simulink model "fourBebop_circle"  (R2017b)
settings: Solver=FixedStepAuto  StartTime=0.0  StopTime=inf  FixedStep=sampleTime  RelTol=1e-3  EnableMultiTasking=on
undefined symbols (not defined in the file or in its folder): Angular, Linear, R
libraries: simulink x20, robotlib x20
(part 1 of 2)
settings Model: Creator=exbot  LastModifiedBy=root
settings DataIOCC: LimitDataPoints=on
settings OptimizationCC: LifeSpan=inf  MaxStackSize=64
settings DebuggingCC: ParameterTunabilityLossMsg=error  AllowSymbolicDim=off  SFUnexpectedBacktrackingDiag=warning  SFNoUnconditionalDefaultTransitionDiag=warning  SFExecutionAtInitializationDiag=none
settings HardwareCC: ProdBitPerPointer=32  ProdBitPerSizeT=32  ProdBitPerPtrDiffT=32  ProdLargestAtomicFloat=None  ProdIntDivRoundTo=Undefined  ProdEndianess=Unspecified  ProdWordSize=32  ProdHWDeviceType=Generic->Unspecified (assume 32-bit Generic)
settings ModelReferenceCC: PropagateSignalLabelsOutOfModel=off
settings SFSimCC: MATLABDynamicMemAlloc=off
settings RTWCC: SystemTargetFile=ert.tlc  HardwareBoard=Robot Operating System (ROS)  TemplateMakefile=ert_default_tmf  Toolchain=Catkin  TargetLang=C++
settings CodeAppCC: ForceParamTrailComments=on  IgnoreCustomStorageClasses=off  OperatorAnnotations=on  SimulinkDataObjDesc=on  SFDataObjDesc=on  MATLABFcnDesc=on  InsertBlockDesc=on  StateflowObjectComments=on  MATLABSourceComments=on
settings ERTTargetCC: MultiwordLength=2048  SupportContinuousTime=on
settings ConfigComp: CovMetricSettings=dw  CovHtmlReporting=on  CovSaveCumulativeToWorkspaceVar=on  CovSaveSingleToWorkspaceVar=on  CovExternalEMLEnable=off

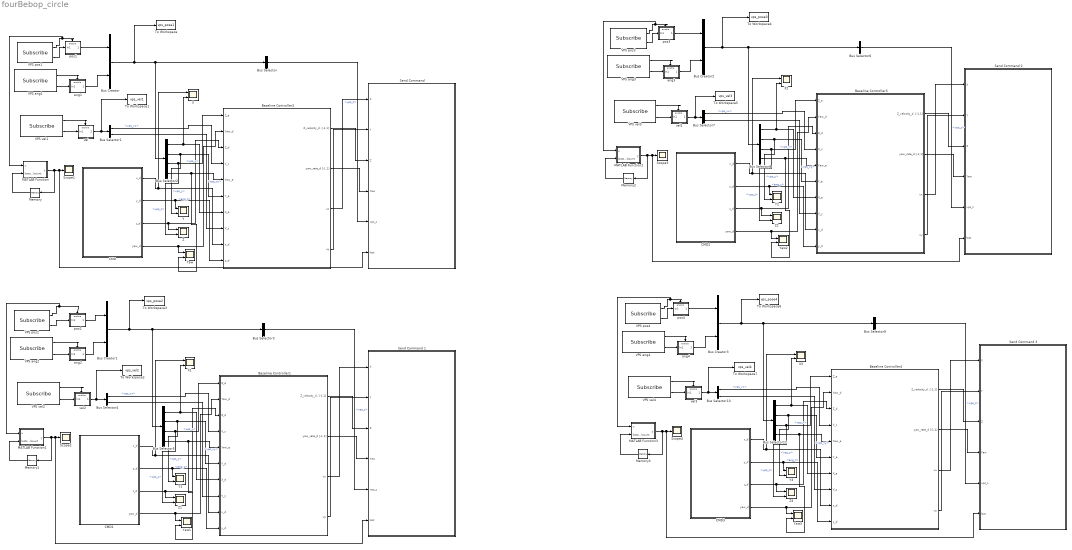
== system fourBebop_circle ==
  Baseline Controller1 : Subsystem  AncestorBlock=ARBlocks/Baseline Controller
  Baseline Controller2 : Subsystem  AncestorBlock=ARBlocks/Baseline Controller
  Baseline Controller3 : Subsystem  AncestorBlock=ARBlocks/Baseline Controller
  Baseline Controller4 : Subsystem  AncestorBlock=ARBlocks/Baseline Controller
  Bus Creator{,1..3} (4 alike) : BusCreator  Inputs=2
  Bus Selector{,3,6,9} (4 alike) : BusSelector  OutputSignals=signal1.vps_z
  Bus Selector{1,4,7,10} (4 alike) : BusSelector  OutputSignals=vps_vx,vps_vy
  Bus Selector{2,5,8,11} (4 alike) : BusSelector  OutputSignals=signal1.vps_x,signal1.vps_y,signal1.vps_z,signal2.ang_z
  CMD : Subsystem
  CMD1 : Subsystem
  CMD2 : Subsystem
  CMD3 : Subsystem
  MATLAB Function : MATLAB Function  TreatAsAtomicUnit=on
  MATLAB Function1 : MATLAB Function  TreatAsAtomicUnit=on
  MATLAB Function2 : MATLAB Function  TreatAsAtomicUnit=on
  MATLAB Function3 : MATLAB Function  TreatAsAtomicUnit=on
  Memory{,1..3} (4 alike) : Memory
  Scope{1..4} (4 alike) : Scope
  "Send Command " : Subsystem
  Send Command 1 : Subsystem
  Send Command 2 : Subsystem
  Send Command 3 : Subsystem
  To Workspace : ToWorkspace  VariableName=vps_pose1  SaveFormat=Timeseries  SampleTime=-1
  To Workspace1 : ToWorkspace  VariableName=vps_vel1  SaveFormat=Timeseries  SampleTime=-1
  To Workspace2 : ToWorkspace  VariableName=vps_vel2  SaveFormat=Timeseries  SampleTime=-1
  To Workspace3 : ToWorkspace  VariableName=vps_pose2  SaveFormat=Timeseries  SampleTime=-1
  To Workspace4 : ToWorkspace  VariableName=vps_pose3  SaveFormat=Timeseries  SampleTime=-1
  To Workspace5 : ToWorkspace  VariableName=vps_vel3  SaveFormat=Timeseries  SampleTime=-1
  To Workspace6 : ToWorkspace  VariableName=vps_pose4  SaveFormat=Timeseries  SampleTime=-1
  To Workspace7 : ToWorkspace  VariableName=vps_vel4  SaveFormat=Timeseries  SampleTime=-1
  VPS ang1 : robotlib/Subscribe  SourceLibraryInfo=This block requires Robotics System Toolbox  topicSource=Select from ROS network  topic=/vps_ang1  messageType=geometry_msgs/PointStamped  sampleTime=-1  messageQueueLength=1
      settings: SourceProductBaseCode=RO
  VPS ang2 : robotlib/Subscribe  SourceLibraryInfo=This block requires Robotics System Toolbox  topicSource=Specify your own  topic=/vps_ang2  messageType=geometry_msgs/PointStamped  sampleTime=-1  messageQueueLength=1
      settings: SourceProductBaseCode=RO
  VPS ang3 : robotlib/Subscribe  SourceLibraryInfo=This block requires Robotics System Toolbox  topicSource=Specify your own  topic=/vps_ang3  messageType=geometry_msgs/PointStamped  sampleTime=-1  messageQueueLength=1
      settings: SourceProductBaseCode=RO
  VPS ang4 : robotlib/Subscribe  SourceLibraryInfo=This block requires Robotics System Toolbox  topicSource=Specify your own  topic=/vps_ang4  messageType=geometry_msgs/PointStamped  sampleTime=-1  messageQueueLength=1
      settings: SourceProductBaseCode=RO
  VPS pos1 : robotlib/Subscribe  SourceLibraryInfo=This block requires Robotics System Toolbox  topicSource=Select from ROS network  topic=/vps_pos1  messageType=geometry_msgs/PointStamped  sampleTime=-1  messageQueueLength=1
      settings: SourceProductBaseCode=RO
  VPS pos2 : robotlib/Subscribe  SourceLibraryInfo=This block requires Robotics System Toolbox  topicSource=Specify your own  topic=/vps_pos2  messageType=geometry_msgs/PointStamped  sampleTime=-1  messageQueueLength=1
      settings: SourceProductBaseCode=RO
  VPS pos3 : robotlib/Subscribe  SourceLibraryInfo=This block requires Robotics System Toolbox  topicSource=Specify your own  topic=/vps_pos3  messageType=geometry_msgs/PointStamped  sampleTime=-1  messageQueueLength=1
      settings: SourceProductBaseCode=RO
  VPS pos4 : robotlib/Subscribe  SourceLibraryInfo=This block requires Robotics System Toolbox  topicSource=Specify your own  topic=/vps_pos4  messageType=geometry_msgs/PointStamped  sampleTime=-1  messageQueueLength=1
      settings: SourceProductBaseCode=RO
  VPS vel1 : robotlib/Subscribe  SourceLibraryInfo=This block requires Robotics System Toolbox  topicSource=Select from ROS network  topic=/vps_vel1  messageType=geometry_msgs/TwistStamped  sampleTime=-1  messageQueueLength=1
      settings: SourceProductBaseCode=RO
  VPS vel2 : robotlib/Subscribe  SourceLibraryInfo=This block requires Robotics System Toolbox  topicSource=Specify your own  topic=/vps_vel2  messageType=geometry_msgs/TwistStamped  sampleTime=-1  messageQueueLength=1
      settings: SourceProductBaseCode=RO
  VPS vel3 : robotlib/Subscribe  SourceLibraryInfo=This block requires Robotics System Toolbox  topicSource=Specify your own  topic=/vps_vel3  messageType=geometry_msgs/TwistStamped  sampleTime=-1  messageQueueLength=1
      settings: SourceProductBaseCode=RO
  VPS vel4 : robotlib/Subscribe  SourceLibraryInfo=This block requires Robotics System Toolbox  topicSource=Specify your own  topic=/vps_vel4  messageType=geometry_msgs/TwistStamped  sampleTime=-1  messageQueueLength=1
      settings: SourceProductBaseCode=RO
  X{,1..3} (4 alike) : Scope  NumInputPorts=2
  Y{,1..3} (4 alike) : Scope  NumInputPorts=2
  Yaw{,1..3} (4 alike) : Scope  NumInputPorts=2
  Z{,1..3} (4 alike) : Scope  NumInputPorts=2
  ang1 : Subsystem
  ang2 : Subsystem
  ang3 : Subsystem
  ang4 : Subsystem
  pos1 : Subsystem
  pos2 : Subsystem
  pos3 : Subsystem
  pos4 : Subsystem
  vel : Subsystem
  vel1 : Subsystem
  vel2 : Subsystem
  vel3 : Subsystem
  wires:
  Bus Creator/1 -> To Workspace/1, Bus Selector2/1, Bus Selector/1
  vel/1(Out1) -> To Workspace1/1, Bus Selector1/1
  Baseline Controller2/3(ux) -> "Send Command "/1(X)
  Baseline Controller2/4(uy) -> "Send Command "/2(Y)
  Baseline Controller2/1(Z_velocity_d. [-1,1]) -> "Send Command "/3(Z)
  Baseline Controller2/2(yaw_rate_d [-1,1]) -> "Send Command "/4(Yaw)
  VPS ang1/1 -> ang1/Enable
  pos1/1(Out1) -> Bus Creator/1
  VPS ang1/2 -> ang1/1(In1)
  VPS pos1/2 -> pos1/1(In1)
  ang1/1(Out1) -> Bus Creator/2
  VPS vel1/1 -> vel/Enable
  VPS vel1/2 -> vel/1(In1)
  Bus Selector/1 -> "Send Command "/5(vps_z)  "<vps_z>"
  Memory/1 -> MATLAB Function/2(lostsigalcount)
  VPS pos1/1 -> MATLAB Function/1(u), pos1/Enable
  MATLAB Function/1(y) -> Memory/1, "Send Command "/6(lost), Scope1/1
  Bus Selector1/1 -> Baseline Controller2/4(" V_x")  "<vps_vx>"
  Bus Selector1/2 -> Baseline Controller2/8(V_y)  "<vps_vy>"
  Bus Selector2/4 -> Yaw/2, Baseline Controller2/5(Yaw_e)  "<ang_z>"
  Bus Selector2/1 -> X/2, Baseline Controller2/7(X_e)  "<vps_x>"
  Bus Selector2/2 -> Y/2, Baseline Controller2/6(Y_e)  "<vps_y>"
  Bus Selector2/3 -> Z/2, Baseline Controller2/1(" Z_e ")  "<vps_z>"
  CMD/4(yaw_d) -> Yaw/1, Baseline Controller2/2(Yaw_d)
  CMD/3(z_d) -> Z/1, Baseline Controller2/3(Z_d)
  CMD/2(y_d) -> Y/1, Baseline Controller2/10(y_d)
  CMD/1(x_d) -> X/1, Baseline Controller2/9(x_d)
  VPS pos2/1 -> MATLAB Function1/1(u), pos2/Enable
  Bus Selector5/2 -> Y1/2, Baseline Controller1/6(Y_e)  "<vps_y>"
  CMD1/1(x_d) -> X1/1, Baseline Controller1/9(x_d)
  Bus Selector3/1 -> Send Command 1/5(vps_z)  "<vps_z>"
  CMD1/2(y_d) -> Y1/1, Baseline Controller1/10(y_d)
  ang2/1(Out1) -> Bus Creator1/2
  Bus Selector5/1 -> X1/2, Baseline Controller1/7(X_e)  "<vps_x>"
  Baseline Controller1/4(uy) -> Send Command 1/2(Y)
  VPS ang2/1 -> ang2/Enable
  Baseline Controller1/2(yaw_rate_d [-1,1]) -> Send Command 1/4(Yaw)
  VPS pos2/2 -> pos2/1(In1)
  vel2/1(Out1) -> To Workspace2/1, Bus Selector4/1
  Bus Selector4/1 -> Baseline Controller1/4(" V_x")  "<vps_vx>"
  Bus Selector4/2 -> Baseline Controller1/8(V_y)  "<vps_vy>"
  Bus Selector5/3 -> Z1/2, Baseline Controller1/1(" Z_e ")  "<vps_z>"
  CMD1/4(yaw_d) -> Yaw1/1, Baseline Controller1/2(Yaw_d)
  pos2/1(Out1) -> Bus Creator1/1
  VPS vel2/2 -> vel2/1(In1)
  VPS vel2/1 -> vel2/Enable
  Bus Creator1/1 -> To Workspace3/1, Bus Selector5/1, Bus Selector3/1
  Bus Selector5/4 -> Yaw1/2, Baseline Controller1/5(Yaw_e)  "<ang_z>"
  VPS ang2/2 -> ang2/1(In1)
  Baseline Controller1/3(ux) -> Send Command 1/1(X)
  Baseline Controller1/1(Z_velocity_d. [-1,1]) -> Send Command 1/3(Z)
  CMD1/3(z_d) -> Z1/1, Baseline Controller1/3(Z_d)
  MATLAB Function1/1(y) -> Memory1/1, Send Command 1/6(lost), Scope2/1
  Memory1/1 -> MATLAB Function1/2(lostsigalcount)
  VPS pos3/1 -> MATLAB Function2/1(u), pos3/Enable
  VPS ang3/2 -> ang3/1(In1)
  Bus Selector6/1 -> Send Command 2/5(vps_z)  "<vps_z>"
  pos3/1(Out1) -> Bus Creator2/1
  Bus Selector7/1 -> Baseline Controller3/4(" V_x")  "<vps_vx>"
  Bus Selector8/4 -> Yaw2/2, Baseline Controller3/5(Yaw_e)  "<ang_z>"
  vel1/1(Out1) -> To Workspace5/1, Bus Selector7/1
  Bus Selector8/3 -> Z2/2, Baseline Controller3/1(" Z_e ")  "<vps_z>"
  VPS pos3/2 -> pos3/1(In1)
  Baseline Controller3/2(yaw_rate_d [-1,1]) -> Send Command 2/4(Yaw)
  CMD2/3(z_d) -> Z2/1, Baseline Controller3/3(Z_d)
  Baseline Controller3/4(uy) -> Send Command 2/2(Y)
  Memory2/1 -> MATLAB Function2/2(lostsigalcount)
  Bus Selector8/1 -> X2/2, Baseline Controller3/7(X_e)  "<vps_x>"
  Bus Creator2/1 -> To Workspace4/1, Bus Selector8/1, Bus Selector6/1
  CMD2/2(y_d) -> Y2/1, Baseline Controller3/10(y_d)
  Bus Selector7/2 -> Baseline Controller3/8(V_y)  "<vps_vy>"
  VPS ang3/1 -> ang3/Enable
  Baseline Controller3/3(ux) -> Send Command 2/1(X)
  Baseline Controller3/1(Z_velocity_d. [-1,1]) -> Send Command 2/3(Z)
  VPS vel3/2 -> vel1/1(In1)
  VPS vel3/1 -> vel1/Enable
  ang3/1(Out1) -> Bus Creator2/2
  MATLAB Function2/1(y) -> Memory2/1, Send Command 2/6(lost), Scope3/1
  CMD2/4(yaw_d) -> Yaw2/1, Baseline Controller3/2(Yaw_d)
  CMD2/1(x_d) -> X2/1, Baseline Controller3/9(x_d)
  Bus Selector8/2 -> Y2/2, Baseline Controller3/6(Y_e)  "<vps_y>"
  Bus Selector10/1 -> Baseline Controller4/4(" V_x")  "<vps_vx>"
  VPS vel4/2 -> vel3/1(In1)
  CMD3/3(z_d) -> Z3/1, Baseline Controller4/3(Z_d)
  Bus Creator3/1 -> To Workspace6/1, Bus Selector11/1, Bus Selector9/1
  Bus Selector11/4 -> Yaw3/2, Baseline Controller4/5(Yaw_e)  "<ang_z>"
  CMD3/4(yaw_d) -> Yaw3/1, Baseline Controller4/2(Yaw_d)
  VPS pos4/1 -> MATLAB Function3/1(u), pos4/Enable
  Baseline Controller4/2(yaw_rate_d [-1,1]) -> Send Command 3/4(Yaw)
  Baseline Controller4/1(Z_velocity_d. [-1,1]) -> Send Command 3/3(Z)
  Bus Selector10/2 -> Baseline Controller4/8(V_y)  "<vps_vy>"
  ang4/1(Out1) -> Bus Creator3/2
  VPS pos4/2 -> pos4/1(In1)
  Memory3/1 -> MATLAB Function3/2(lostsigalcount)
  Baseline Controller4/3(ux) -> Send Command 3/1(X)
  Bus Selector11/1 -> X3/2, Baseline Controller4/7(X_e)  "<vps_x>"
  MATLAB Function3/1(y) -> Memory3/1, Send Command 3/6(lost), Scope4/1
  VPS vel4/1 -> vel3/Enable
  CMD3/2(y_d) -> Y3/1, Baseline Controller4/10(y_d)
  Bus Selector11/2 -> Y3/2, Baseline Controller4/6(Y_e)  "<vps_y>"
  Bus Selector11/3 -> Z3/2, Baseline Controller4/1(" Z_e ")  "<vps_z>"
  Baseline Controller4/4(uy) -> Send Command 3/2(Y)
  VPS ang4/2 -> ang4/1(In1)
  vel3/1(Out1) -> To Workspace7/1, Bus Selector10/1
  VPS ang4/1 -> ang4/Enable
  pos4/1(Out1) -> Bus Creator3/1
  CMD3/1(x_d) -> X3/1, Baseline Controller4/9(x_d)
  Bus Selector9/1 -> Send Command 3/5(vps_z)  "<vps_z>"

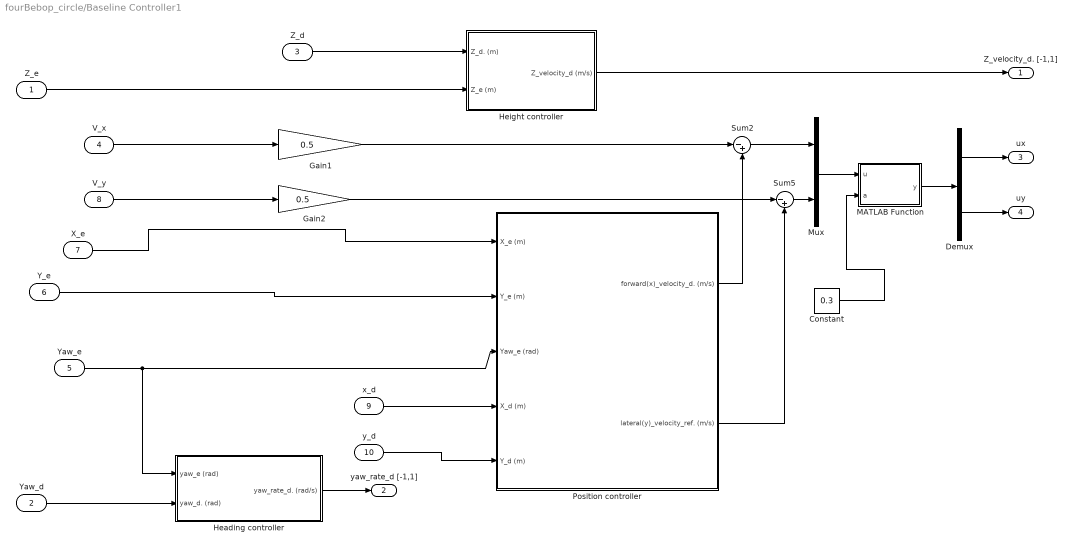
== system fourBebop_circle/Baseline Controller1 ==
  " Z_e " : Inport
  Yaw_d : Inport  Port=2
  Z_d : Inport  Port=3
  " V_x" : Inport  Port=4
  Yaw_e : Inport  Port=5
  Y_e : Inport  Port=6
  X_e : Inport  Port=7
  V_y : Inport  Port=8
  x_d : Inport  Port=9
  y_d : Inport  Port=10
  Constant : Constant  Value=0.3
  Demux : Demux  Outputs=2
  Gain1 : Gain  Gain=0.5
  Gain2 : Gain  Gain=0.5
  Heading controller : Subsystem
  "Height controller " : Subsystem
  MATLAB Function : MATLAB Function  TreatAsAtomicUnit=on
  Mux : Mux  Inputs=2
  Position controller : Subsystem
  Sum2 : Sum  Inputs=|-+
  Sum5 : Sum  Inputs=|-+
  Z_velocity_d. [-1,1] : Outport
  yaw_rate_d [-1,1] : Outport  Port=2
  ux : Outport  Port=3
  uy : Outport  Port=4
  wires:
  Position controller/2(lateral(y)_velocity_ref. (m/s)) -> Sum5/2
  Gain2/1 -> Sum5/1
  V_y/1 -> Gain2/1
  Position controller/1(forward(x)_velocity_d. (m/s)) -> Sum2/2
  Gain1/1 -> Sum2/1
  Yaw_e/1 -> Heading controller/1(yaw_e (rad)), Position controller/3(Yaw_e (rad))
  " Z_e "/1 -> "Height controller "/2(Z_e (m))
  "Height controller "/1(Z_velocity_d (m/s)) -> Z_velocity_d. [-1,1]/1
  " V_x"/1 -> Gain1/1
  Heading controller/1(yaw_rate_d. (rad/s)) -> yaw_rate_d [-1,1]/1
  X_e/1 -> Position controller/1(X_e (m))
  Y_e/1 -> Position controller/2(Y_e (m))
  Sum2/1 -> Mux/1
  Sum5/1 -> Mux/2
  Yaw_d/1 -> Heading controller/2(yaw_d. (rad))
  Mux/1 -> MATLAB Function/1(u)
  MATLAB Function/1(y) -> Demux/1
  Demux/1 -> ux/1
  Demux/2 -> uy/1
  Constant/1 -> MATLAB Function/2(a)
  Z_d/1 -> "Height controller "/1(Z_d. (m))
  x_d/1 -> Position controller/4(X_d (m))
  y_d/1 -> Position controller/5(Y_d (m))

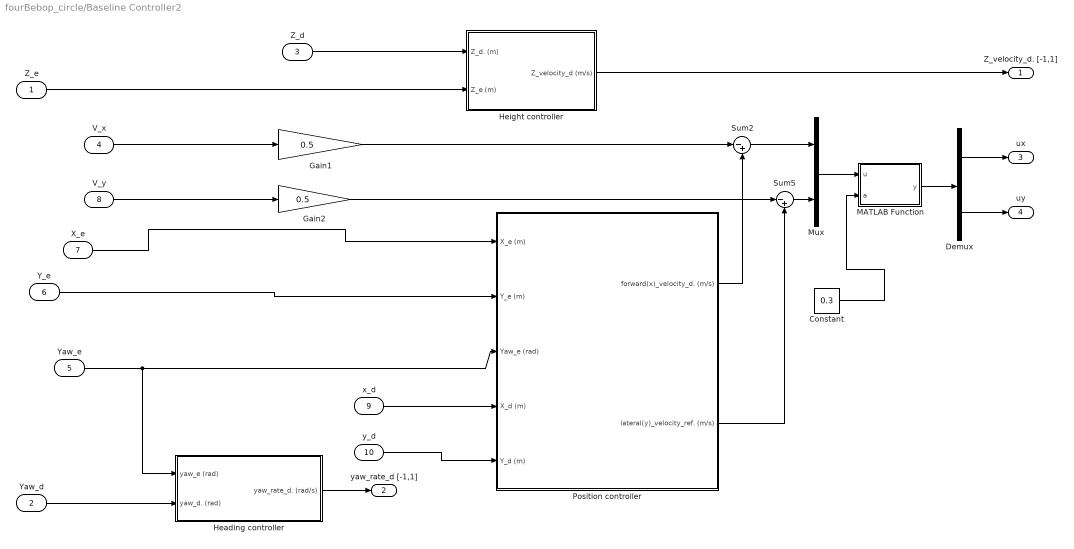
== system fourBebop_circle/Baseline Controller2 ==
  " Z_e " : Inport
  Yaw_d : Inport  Port=2
  Z_d : Inport  Port=3
  " V_x" : Inport  Port=4
  Yaw_e : Inport  Port=5
  Y_e : Inport  Port=6
  X_e : Inport  Port=7
  V_y : Inport  Port=8
  x_d : Inport  Port=9
  y_d : Inport  Port=10
  Constant : Constant  Value=0.3
  Demux : Demux  Outputs=2
  Gain1 : Gain  Gain=0.5
  Gain2 : Gain  Gain=0.5
  Heading controller : Subsystem
  "Height controller " : Subsystem
  MATLAB Function : MATLAB Function  TreatAsAtomicUnit=on
  Mux : Mux  Inputs=2
  Position controller : Subsystem
  Sum2 : Sum  Inputs=|-+
  Sum5 : Sum  Inputs=|-+
  Z_velocity_d. [-1,1] : Outport
  yaw_rate_d [-1,1] : Outport  Port=2
  ux : Outport  Port=3
  uy : Outport  Port=4
  wires:
  Position controller/2(lateral(y)_velocity_ref. (m/s)) -> Sum5/2
  Gain2/1 -> Sum5/1
  V_y/1 -> Gain2/1
  Position controller/1(forward(x)_velocity_d. (m/s)) -> Sum2/2
  Gain1/1 -> Sum2/1
  Yaw_e/1 -> Heading controller/1(yaw_e (rad)), Position controller/3(Yaw_e (rad))
  " Z_e "/1 -> "Height controller "/2(Z_e (m))
  "Height controller "/1(Z_velocity_d (m/s)) -> Z_velocity_d. [-1,1]/1
  " V_x"/1 -> Gain1/1
  Heading controller/1(yaw_rate_d. (rad/s)) -> yaw_rate_d [-1,1]/1
  X_e/1 -> Position controller/1(X_e (m))
  Y_e/1 -> Position controller/2(Y_e (m))
  Sum2/1 -> Mux/1
  Sum5/1 -> Mux/2
  Yaw_d/1 -> Heading controller/2(yaw_d. (rad))
  Mux/1 -> MATLAB Function/1(u)
  MATLAB Function/1(y) -> Demux/1
  Demux/1 -> ux/1
  Demux/2 -> uy/1
  Constant/1 -> MATLAB Function/2(a)
  Z_d/1 -> "Height controller "/1(Z_d. (m))
  x_d/1 -> Position controller/4(X_d (m))
  y_d/1 -> Position controller/5(Y_d (m))

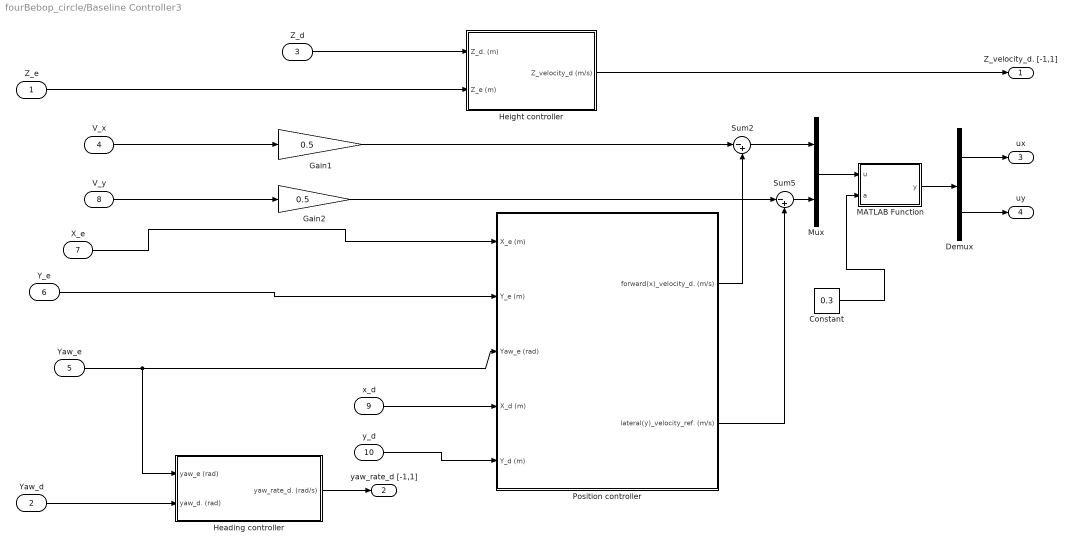
== system fourBebop_circle/Baseline Controller3 ==
  " Z_e " : Inport
  Yaw_d : Inport  Port=2
  Z_d : Inport  Port=3
  " V_x" : Inport  Port=4
  Yaw_e : Inport  Port=5
  Y_e : Inport  Port=6
  X_e : Inport  Port=7
  V_y : Inport  Port=8
  x_d : Inport  Port=9
  y_d : Inport  Port=10
  Constant : Constant  Value=0.3
  Demux : Demux  Outputs=2
  Gain1 : Gain  Gain=0.5
  Gain2 : Gain  Gain=0.5
  Heading controller : Subsystem
  "Height controller " : Subsystem
  MATLAB Function : MATLAB Function  TreatAsAtomicUnit=on
  Mux : Mux  Inputs=2
  Position controller : Subsystem
  Sum2 : Sum  Inputs=|-+
  Sum5 : Sum  Inputs=|-+
  Z_velocity_d. [-1,1] : Outport
  yaw_rate_d [-1,1] : Outport  Port=2
  ux : Outport  Port=3
  uy : Outport  Port=4
  wires:
  Position controller/2(lateral(y)_velocity_ref. (m/s)) -> Sum5/2
  Gain2/1 -> Sum5/1
  V_y/1 -> Gain2/1
  Position controller/1(forward(x)_velocity_d. (m/s)) -> Sum2/2
  Gain1/1 -> Sum2/1
  Yaw_e/1 -> Heading controller/1(yaw_e (rad)), Position controller/3(Yaw_e (rad))
  " Z_e "/1 -> "Height controller "/2(Z_e (m))
  "Height controller "/1(Z_velocity_d (m/s)) -> Z_velocity_d. [-1,1]/1
  " V_x"/1 -> Gain1/1
  Heading controller/1(yaw_rate_d. (rad/s)) -> yaw_rate_d [-1,1]/1
  X_e/1 -> Position controller/1(X_e (m))
  Y_e/1 -> Position controller/2(Y_e (m))
  Sum2/1 -> Mux/1
  Sum5/1 -> Mux/2
  Yaw_d/1 -> Heading controller/2(yaw_d. (rad))
  Mux/1 -> MATLAB Function/1(u)
  MATLAB Function/1(y) -> Demux/1
  Demux/1 -> ux/1
  Demux/2 -> uy/1
  Constant/1 -> MATLAB Function/2(a)
  Z_d/1 -> "Height controller "/1(Z_d. (m))
  x_d/1 -> Position controller/4(X_d (m))
  y_d/1 -> Position controller/5(Y_d (m))

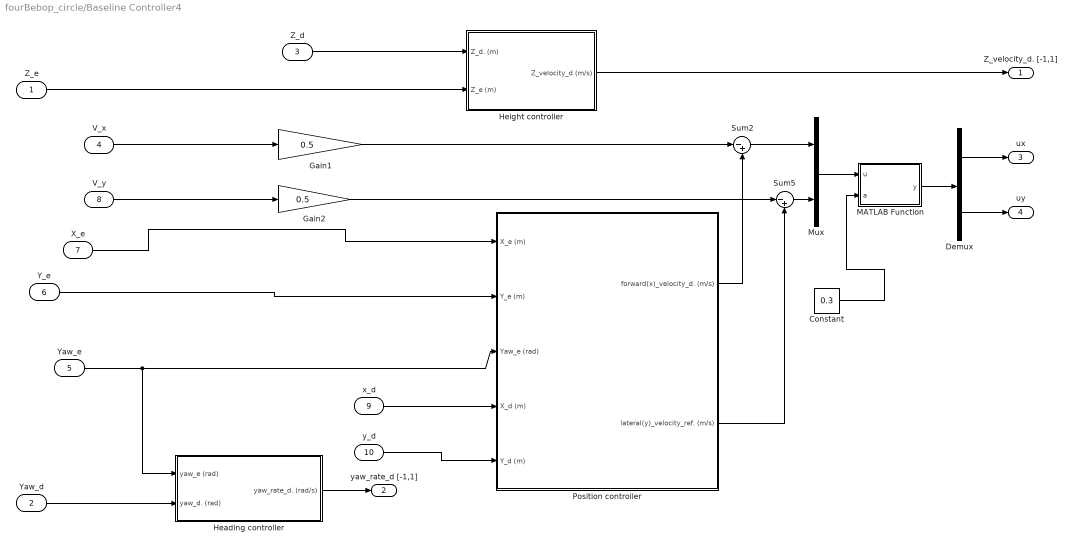
== system fourBebop_circle/Baseline Controller4 ==
  " Z_e " : Inport
  Yaw_d : Inport  Port=2
  Z_d : Inport  Port=3
  " V_x" : Inport  Port=4
  Yaw_e : Inport  Port=5
  Y_e : Inport  Port=6
  X_e : Inport  Port=7
  V_y : Inport  Port=8
  x_d : Inport  Port=9
  y_d : Inport  Port=10
  Constant : Constant  Value=0.3
  Demux : Demux  Outputs=2
  Gain1 : Gain  Gain=0.5
  Gain2 : Gain  Gain=0.5
  Heading controller : Subsystem
  "Height controller " : Subsystem
  MATLAB Function : MATLAB Function  TreatAsAtomicUnit=on
  Mux : Mux  Inputs=2
  Position controller : Subsystem
  Sum2 : Sum  Inputs=|-+
  Sum5 : Sum  Inputs=|-+
  Z_velocity_d. [-1,1] : Outport
  yaw_rate_d [-1,1] : Outport  Port=2
  ux : Outport  Port=3
  uy : Outport  Port=4
  wires:
  Position controller/2(lateral(y)_velocity_ref. (m/s)) -> Sum5/2
  Gain2/1 -> Sum5/1
  V_y/1 -> Gain2/1
  Position controller/1(forward(x)_velocity_d. (m/s)) -> Sum2/2
  Gain1/1 -> Sum2/1
  Yaw_e/1 -> Heading controller/1(yaw_e (rad)), Position controller/3(Yaw_e (rad))
  " Z_e "/1 -> "Height controller "/2(Z_e (m))
  "Height controller "/1(Z_velocity_d (m/s)) -> Z_velocity_d. [-1,1]/1
  " V_x"/1 -> Gain1/1
  Heading controller/1(yaw_rate_d. (rad/s)) -> yaw_rate_d [-1,1]/1
  X_e/1 -> Position controller/1(X_e (m))
  Y_e/1 -> Position controller/2(Y_e (m))
  Sum2/1 -> Mux/1
  Sum5/1 -> Mux/2
  Yaw_d/1 -> Heading controller/2(yaw_d. (rad))
  Mux/1 -> MATLAB Function/1(u)
  MATLAB Function/1(y) -> Demux/1
  Demux/1 -> ux/1
  Demux/2 -> uy/1
  Constant/1 -> MATLAB Function/2(a)
  Z_d/1 -> "Height controller "/1(Z_d. (m))
  x_d/1 -> Position controller/4(X_d (m))
  y_d/1 -> Position controller/5(Y_d (m))

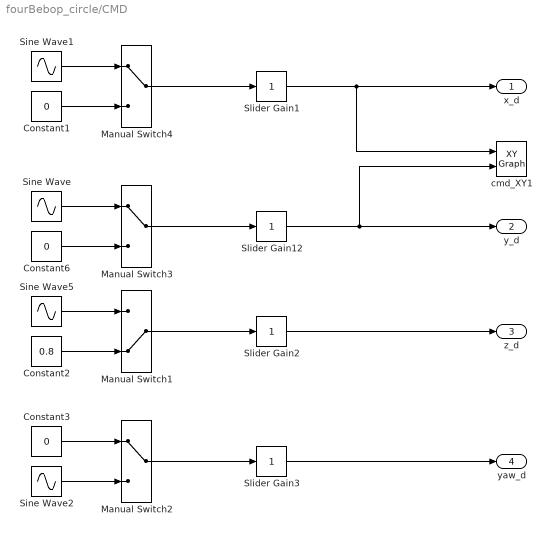
== system fourBebop_circle/CMD ==
  Constant1 : Constant  Value=0
  Constant2 : Constant  Value=0.8
  Constant3 : Constant  Value=0
  Constant6 : Constant  Value=0
  Manual Switch1 : ManualSwitch  CurrentSetting=0
  Manual Switch2 : ManualSwitch
  Manual Switch3 : ManualSwitch
  Manual Switch4 : ManualSwitch
  Sine Wave : Sin  Amplitude=R  Frequency=0.3
  Sine Wave1 : Sin  Amplitude=R  Frequency=0.3  Phase=pi/2
  Sine Wave2 : Sin  Amplitude=0.3
  Sine Wave5 : Sin  Amplitude=0.4  Frequency=2
  Slider Gain1 : simulink/Math Operations/Slider Gain  gain=1  low=-2  high=2
  Slider Gain12 : simulink/Math Operations/Slider Gain  gain=1  low=-2  high=2
  Slider Gain2 : simulink/Math Operations/Slider Gain  gain=1  low=-2  high=2
  Slider Gain3 : simulink/Math Operations/Slider Gain  gain=1  low=0  high=2
  cmd_XY1 : simulink/Sinks/XY Graph  xmin=-2  xmax=2  ymin=-2  ymax=2  st=-1
  x_d : Outport
  y_d : Outport  Port=2
  z_d : Outport  Port=3
  yaw_d : Outport  Port=4
  wires:
  Sine Wave/1 -> Manual Switch3/1
  Manual Switch3/1 -> Slider Gain12/1
  Constant6/1 -> Manual Switch3/2
  Slider Gain12/1 -> cmd_XY1/2, y_d/1
  Manual Switch1/1 -> Slider Gain2/1
  Constant1/1 -> Manual Switch4/2
  Sine Wave1/1 -> Manual Switch4/1
  Manual Switch4/1 -> Slider Gain1/1
  Slider Gain1/1 -> cmd_XY1/1, x_d/1
  Constant2/1 -> Manual Switch1/2
  Sine Wave5/1 -> Manual Switch1/1
  Manual Switch2/1 -> Slider Gain3/1
  Slider Gain3/1 -> yaw_d/1
  Sine Wave2/1 -> Manual Switch2/2
  Constant3/1 -> Manual Switch2/1
  Slider Gain2/1 -> z_d/1

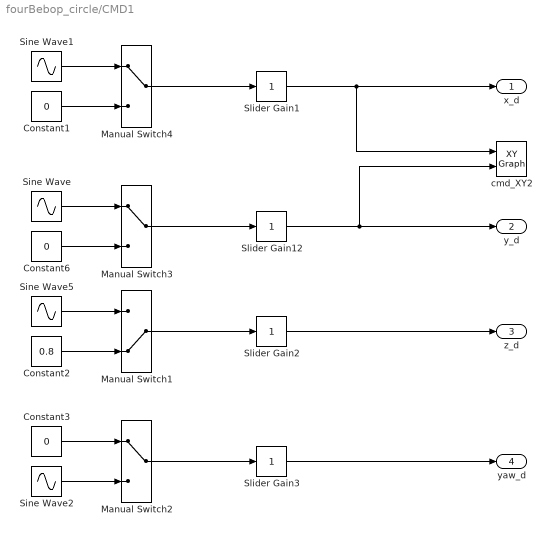
== system fourBebop_circle/CMD1 ==
  Constant1 : Constant  Value=0
  Constant2 : Constant  Value=0.8
  Constant3 : Constant  Value=0
  Constant6 : Constant  Value=0
  Manual Switch1 : ManualSwitch  CurrentSetting=0
  Manual Switch2 : ManualSwitch
  Manual Switch3 : ManualSwitch
  Manual Switch4 : ManualSwitch
  Sine Wave : Sin  Amplitude=R  Frequency=0.3  Phase=2*pi/3
  Sine Wave1 : Sin  Amplitude=R  Frequency=0.3  Phase=7*pi/6
  Sine Wave2 : Sin  Amplitude=0.3
  Sine Wave5 : Sin  Amplitude=0.4  Frequency=2
  Slider Gain1 : simulink/Math Operations/Slider Gain  gain=1  low=-2  high=2
  Slider Gain12 : simulink/Math Operations/Slider Gain  gain=1  low=-2  high=2
  Slider Gain2 : simulink/Math Operations/Slider Gain  gain=1  low=-2  high=2
  Slider Gain3 : simulink/Math Operations/Slider Gain  gain=1  low=0  high=2
  cmd_XY2 : simulink/Sinks/XY Graph  xmin=-2  xmax=2  ymin=-2  ymax=2  st=-1
  x_d : Outport
  y_d : Outport  Port=2
  z_d : Outport  Port=3
  yaw_d : Outport  Port=4
  wires:
  Sine Wave/1 -> Manual Switch3/1
  Manual Switch3/1 -> Slider Gain12/1
  Constant6/1 -> Manual Switch3/2
  Slider Gain12/1 -> cmd_XY2/2, y_d/1
  Manual Switch1/1 -> Slider Gain2/1
  Constant1/1 -> Manual Switch4/2
  Sine Wave1/1 -> Manual Switch4/1
  Manual Switch4/1 -> Slider Gain1/1
  Slider Gain1/1 -> cmd_XY2/1, x_d/1
  Constant2/1 -> Manual Switch1/2
  Sine Wave5/1 -> Manual Switch1/1
  Manual Switch2/1 -> Slider Gain3/1
  Slider Gain3/1 -> yaw_d/1
  Sine Wave2/1 -> Manual Switch2/2
  Constant3/1 -> Manual Switch2/1
  Slider Gain2/1 -> z_d/1

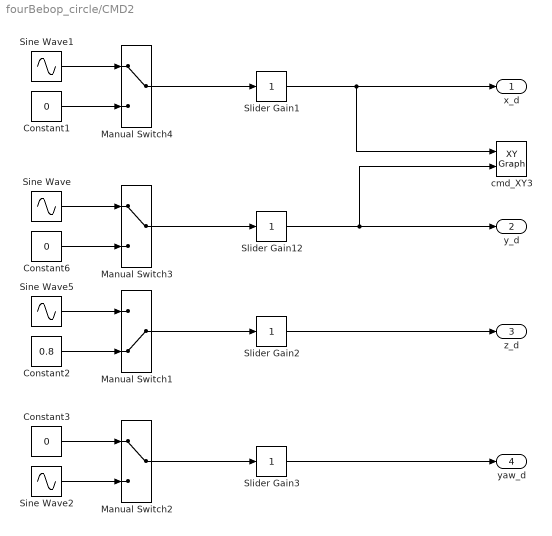
== system fourBebop_circle/CMD2 ==
  Constant1 : Constant  Value=0
  Constant2 : Constant  Value=0.8
  Constant3 : Constant  Value=0
  Constant6 : Constant  Value=0
  Manual Switch1 : ManualSwitch  CurrentSetting=0
  Manual Switch2 : ManualSwitch
  Manual Switch3 : ManualSwitch
  Manual Switch4 : ManualSwitch
  Sine Wave : Sin  Amplitude=R  Frequency=0.3  Phase=4*pi/3
  Sine Wave1 : Sin  Amplitude=R  Frequency=0.3  Phase=11*pi/6
  Sine Wave2 : Sin  Amplitude=0.3
  Sine Wave5 : Sin  Amplitude=0.4  Frequency=2
  Slider Gain1 : simulink/Math Operations/Slider Gain  gain=1  low=-2  high=2
  Slider Gain12 : simulink/Math Operations/Slider Gain  gain=1  low=-2  high=2
  Slider Gain2 : simulink/Math Operations/Slider Gain  gain=1  low=-2  high=2
  Slider Gain3 : simulink/Math Operations/Slider Gain  gain=1  low=0  high=2
  cmd_XY3 : simulink/Sinks/XY Graph  xmin=-2  xmax=2  ymin=-2  ymax=2  st=-1
  x_d : Outport
  y_d : Outport  Port=2
  z_d : Outport  Port=3
  yaw_d : Outport  Port=4
  wires:
  Sine Wave/1 -> Manual Switch3/1
  Manual Switch3/1 -> Slider Gain12/1
  Constant6/1 -> Manual Switch3/2
  Slider Gain12/1 -> cmd_XY3/2, y_d/1
  Manual Switch1/1 -> Slider Gain2/1
  Constant1/1 -> Manual Switch4/2
  Sine Wave1/1 -> Manual Switch4/1
  Manual Switch4/1 -> Slider Gain1/1
  Slider Gain1/1 -> cmd_XY3/1, x_d/1
  Constant2/1 -> Manual Switch1/2
  Sine Wave5/1 -> Manual Switch1/1
  Manual Switch2/1 -> Slider Gain3/1
  Slider Gain3/1 -> yaw_d/1
  Sine Wave2/1 -> Manual Switch2/2
  Constant3/1 -> Manual Switch2/1
  Slider Gain2/1 -> z_d/1

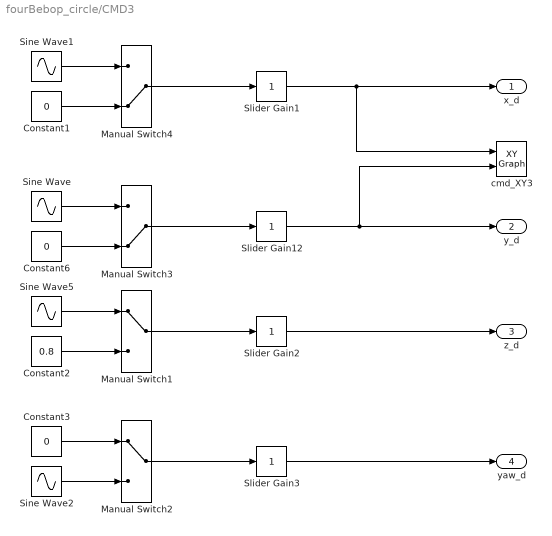
== system fourBebop_circle/CMD3 ==
  Constant1 : Constant  Value=0
  Constant2 : Constant  Value=0.8
  Constant3 : Constant  Value=0
  Constant6 : Constant  Value=0
  Manual Switch1 : ManualSwitch
  Manual Switch2 : ManualSwitch
  Manual Switch3 : ManualSwitch  CurrentSetting=0
  Manual Switch4 : ManualSwitch  CurrentSetting=0
  Sine Wave : Sin  Amplitude=R  Frequency=0.3  Phase=4*pi/3
  Sine Wave1 : Sin  Amplitude=R  Frequency=0.3  Phase=11*pi/6
  Sine Wave2 : Sin  Amplitude=0.3
  Sine Wave5 : Sin  Amplitude=0.2  Bias=1  Frequency=0.2
  Slider Gain1 : simulink/Math Operations/Slider Gain  gain=1  low=-2  high=2
  Slider Gain12 : simulink/Math Operations/Slider Gain  gain=1  low=-2  high=2
  Slider Gain2 : simulink/Math Operations/Slider Gain  gain=1  low=-2  high=2
  Slider Gain3 : simulink/Math Operations/Slider Gain  gain=1  low=0  high=2
  cmd_XY3 : simulink/Sinks/XY Graph  xmin=-2  xmax=2  ymin=-2  ymax=2  st=-1
  x_d : Outport
  y_d : Outport  Port=2
  z_d : Outport  Port=3
  yaw_d : Outport  Port=4
  wires:
  Sine Wave/1 -> Manual Switch3/1
  Manual Switch3/1 -> Slider Gain12/1
  Constant6/1 -> Manual Switch3/2
  Slider Gain12/1 -> cmd_XY3/2, y_d/1
  Manual Switch1/1 -> Slider Gain2/1
  Constant1/1 -> Manual Switch4/2
  Sine Wave1/1 -> Manual Switch4/1
  Manual Switch4/1 -> Slider Gain1/1
  Slider Gain1/1 -> cmd_XY3/1, x_d/1
  Constant2/1 -> Manual Switch1/2
  Sine Wave5/1 -> Manual Switch1/1
  Manual Switch2/1 -> Slider Gain3/1
  Slider Gain3/1 -> yaw_d/1
  Sine Wave2/1 -> Manual Switch2/2
  Constant3/1 -> Manual Switch2/1
  Slider Gain2/1 -> z_d/1

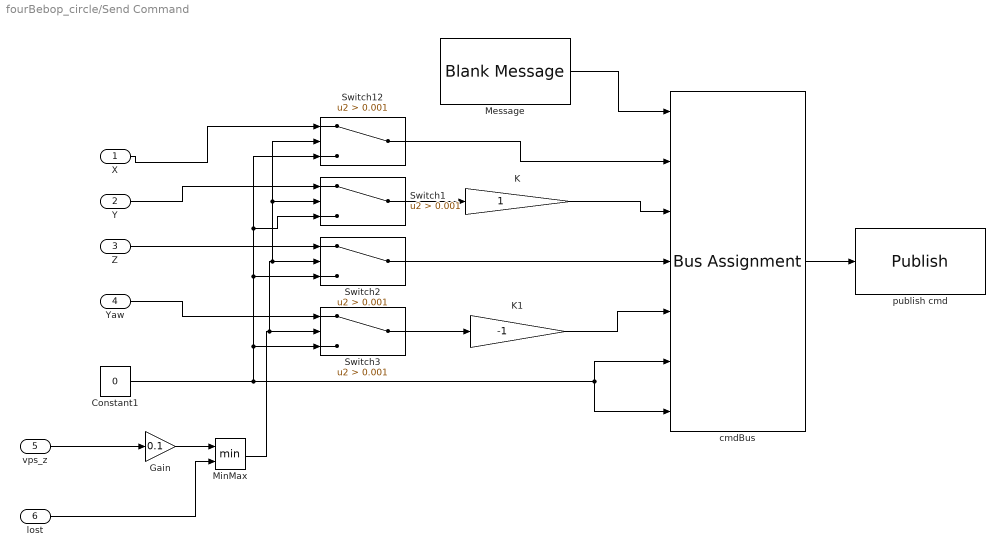
== system fourBebop_circle/Send Command  ==
  X : Inport
  Y : Inport  Port=2
  Z : Inport  Port=3
  Yaw : Inport  Port=4
  vps_z : Inport  Port=5
  lost : Inport  Port=6
  " Message" : robotlib/Blank Message  SourceLibraryInfo=This block requires Robotics System Toolbox  messageType=geometry_msgs/Twist  SampleTime=inf
      settings: SourceProductBaseCode=RO
  Constant1 : Constant  Value=0
  Gain : Gain  Gain=0.1
  K : Gain
  K1 : Gain  Gain=-1
  MinMax : MinMax  Inputs=2
  Switch{1..3,12} (4 alike) : Switch  Criteria=u2 > Threshold  Threshold=0.001
  cmdBus : BusAssignment  AssignedSignals=Linear.X,Linear.Y,Linear.Z,Angular.Z,Angular.X,Angular.Y
  publish cmd : robotlib/Publish  SourceLibraryInfo=This block requires Robotics System Toolbox  topicSource=Select from ROS network  topic=/bebop1/cmd_vel  messageType=geometry_msgs/Twist  messageQueueLength=1
      settings: SourceProductBaseCode=RO
  wires:
  cmdBus/1 -> publish cmd/1
  Constant1/1 -> Switch3/3, Switch2/3, Switch1/3, Switch12/3, cmdBus/6, cmdBus/7
  K/1 -> cmdBus/3
  K1/1 -> cmdBus/5
  " Message"/1 -> cmdBus/1
  Switch12/1 -> cmdBus/2
  X/1 -> Switch12/1
  Switch1/1 -> K/1
  Y/1 -> Switch1/1
  Switch2/1 -> cmdBus/4
  Z/1 -> Switch2/1
  Switch3/1 -> K1/1
  Yaw/1 -> Switch3/1
  vps_z/1 -> Gain/1
  MinMax/1 -> Switch1/2, Switch12/2, Switch2/2, Switch3/2
  Gain/1 -> MinMax/1
  lost/1 -> MinMax/2

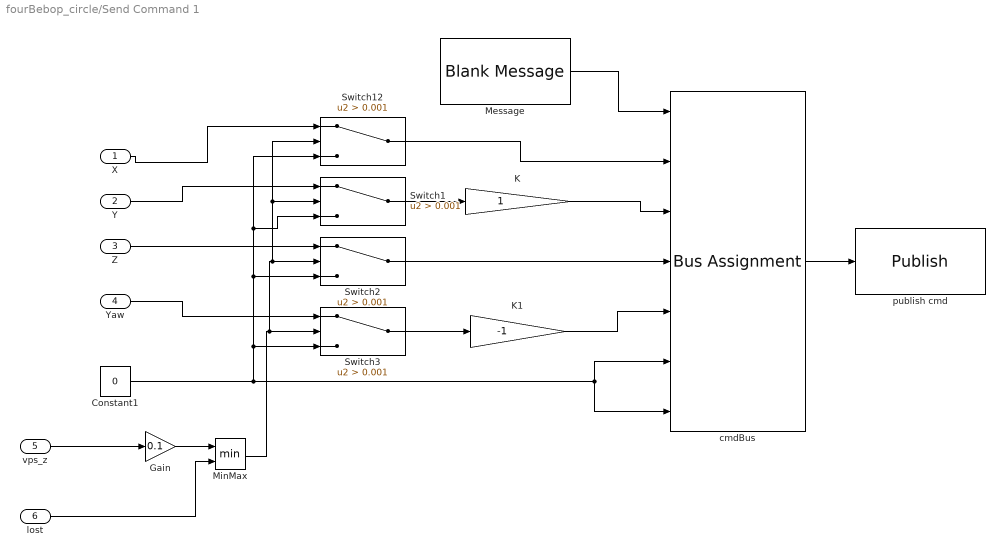
== system fourBebop_circle/Send Command 1 ==
  X : Inport
  Y : Inport  Port=2
  Z : Inport  Port=3
  Yaw : Inport  Port=4
  vps_z : Inport  Port=5
  lost : Inport  Port=6
  " Message" : robotlib/Blank Message  SourceLibraryInfo=This block requires Robotics System Toolbox  messageType=geometry_msgs/Twist  SampleTime=inf
      settings: SourceProductBaseCode=RO
  Constant1 : Constant  Value=0
  Gain : Gain  Gain=0.1
  K : Gain
  K1 : Gain  Gain=-1
  MinMax : MinMax  Inputs=2
  Switch{1..3,12} (4 alike) : Switch  Criteria=u2 > Threshold  Threshold=0.001
  cmdBus : BusAssignment  AssignedSignals=Linear.X,Linear.Y,Linear.Z,Angular.Z,Angular.X,Angular.Y
  publish cmd : robotlib/Publish  SourceLibraryInfo=This block requires Robotics System Toolbox  topicSource=Specify your own  topic=/bebop2/cmd_vel  messageType=geometry_msgs/Twist  messageQueueLength=1
      settings: SourceProductBaseCode=RO
  wires:
  cmdBus/1 -> publish cmd/1
  Constant1/1 -> Switch3/3, Switch2/3, Switch1/3, Switch12/3, cmdBus/6, cmdBus/7
  K/1 -> cmdBus/3
  K1/1 -> cmdBus/5
  " Message"/1 -> cmdBus/1
  Switch12/1 -> cmdBus/2
  X/1 -> Switch12/1
  Switch1/1 -> K/1
  Y/1 -> Switch1/1
  Switch2/1 -> cmdBus/4
  Z/1 -> Switch2/1
  Switch3/1 -> K1/1
  Yaw/1 -> Switch3/1
  vps_z/1 -> Gain/1
  MinMax/1 -> Switch1/2, Switch12/2, Switch2/2, Switch3/2
  Gain/1 -> MinMax/1
  lost/1 -> MinMax/2

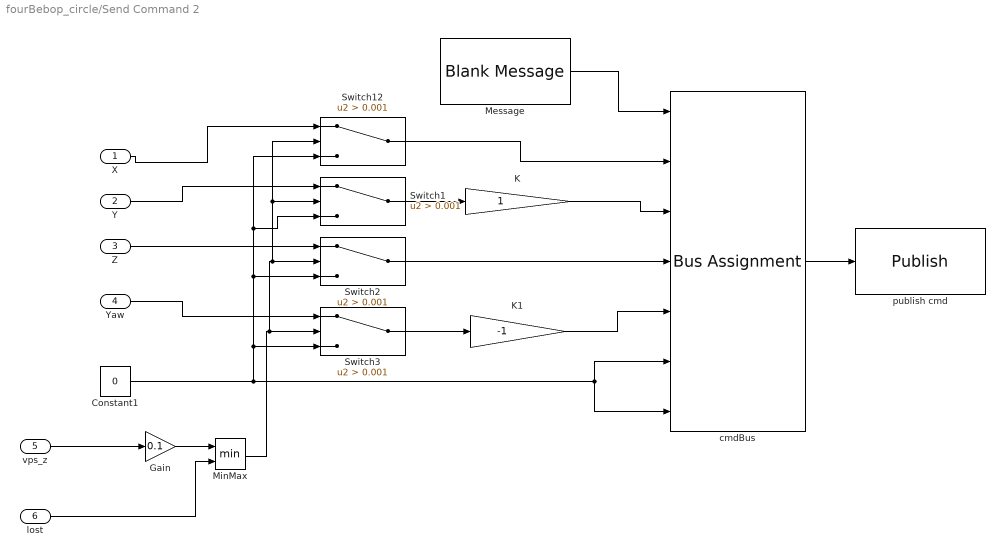
== system fourBebop_circle/Send Command 2 ==
  X : Inport
  Y : Inport  Port=2
  Z : Inport  Port=3
  Yaw : Inport  Port=4
  vps_z : Inport  Port=5
  lost : Inport  Port=6
  " Message" : robotlib/Blank Message  SourceLibraryInfo=This block requires Robotics System Toolbox  messageType=geometry_msgs/Twist  SampleTime=inf
      settings: SourceProductBaseCode=RO
  Constant1 : Constant  Value=0
  Gain : Gain  Gain=0.1
  K : Gain
  K1 : Gain  Gain=-1
  MinMax : MinMax  Inputs=2
  Switch{1..3,12} (4 alike) : Switch  Criteria=u2 > Threshold  Threshold=0.001
  cmdBus : BusAssignment  AssignedSignals=Linear.X,Linear.Y,Linear.Z,Angular.Z,Angular.X,Angular.Y
  publish cmd : robotlib/Publish  SourceLibraryInfo=This block requires Robotics System Toolbox  topicSource=Specify your own  topic=/bebop3/cmd_vel  messageType=geometry_msgs/Twist  messageQueueLength=1
      settings: SourceProductBaseCode=RO
  wires:
  cmdBus/1 -> publish cmd/1
  Constant1/1 -> Switch3/3, Switch2/3, Switch1/3, Switch12/3, cmdBus/6, cmdBus/7
  K/1 -> cmdBus/3
  K1/1 -> cmdBus/5
  " Message"/1 -> cmdBus/1
  Switch12/1 -> cmdBus/2
  X/1 -> Switch12/1
  Switch1/1 -> K/1
  Y/1 -> Switch1/1
  Switch2/1 -> cmdBus/4
  Z/1 -> Switch2/1
  Switch3/1 -> K1/1
  Yaw/1 -> Switch3/1
  vps_z/1 -> Gain/1
  MinMax/1 -> Switch1/2, Switch12/2, Switch2/2, Switch3/2
  Gain/1 -> MinMax/1
  lost/1 -> MinMax/2

== system fourBebop_circle/Send Command 3 ==
  X : Inport
  Y : Inport  Port=2
  Z : Inport  Port=3
  Yaw : Inport  Port=4
  vps_z : Inport  Port=5
  lost : Inport  Port=6
  " Message" : robotlib/Blank Message  SourceLibraryInfo=This block requires Robotics System Toolbox  messageType=geometry_msgs/Twist  SampleTime=inf
      settings: SourceProductBaseCode=RO
  Constant1 : Constant  Value=0
  Gain : Gain  Gain=0.1
  K : Gain
  K1 : Gain  Gain=-1
  MinMax : MinMax  Inputs=2
  Switch{1..3,12} (4 alike) : Switch  Criteria=u2 > Threshold  Threshold=0.001
  cmdBus : BusAssignment  AssignedSignals=Linear.X,Linear.Y,Linear.Z,Angular.Z,Angular.X,Angular.Y
  publish cmd : robotlib/Publish  SourceLibraryInfo=This block requires Robotics System Toolbox  topicSource=Specify your own  topic=/bebop4/cmd_vel  messageType=geometry_msgs/Twist  messageQueueLength=1
      settings: SourceProductBaseCode=RO
  wires:
  cmdBus/1 -> publish cmd/1
  Constant1/1 -> Switch3/3, Switch2/3, Switch1/3, Switch12/3, cmdBus/6, cmdBus/7
  K/1 -> cmdBus/3
  K1/1 -> cmdBus/5
  " Message"/1 -> cmdBus/1
  Switch12/1 -> cmdBus/2
  X/1 -> Switch12/1
  Switch1/1 -> K/1
  Y/1 -> Switch1/1
  Switch2/1 -> cmdBus/4
  Z/1 -> Switch2/1
  Switch3/1 -> K1/1
  Yaw/1 -> Switch3/1
  vps_z/1 -> Gain/1
  MinMax/1 -> Switch1/2, Switch12/2, Switch2/2, Switch3/2
  Gain/1 -> MinMax/1
  lost/1 -> MinMax/2

== system fourBebop_circle/ang1 ==
  In1 : Inport
  Enable : EnablePort
  " " : MATLAB Function  TreatAsAtomicUnit=on
  Bus Creator : BusCreator  Inputs=3
  Bus Selector2 : BusSelector  OutputSignals=Point.X,Point.Y,Point.Z
  Out1 : Outport
  wires:
  Bus Creator/1 -> Out1/1
  In1/1 -> Bus Selector2/1
  Bus Selector2/2 -> " "/2(Y)  "<Y>"
  Bus Selector2/1 -> " "/1(X)  "<X>"
  " "/1(ang_x) -> Bus Creator/1
  " "/2(ang_y) -> Bus Creator/2
  " "/3(ang_z) -> Bus Creator/3
  Bus Selector2/3 -> " "/3(Z)  "<Z>"

== system fourBebop_circle/ang2 ==
  In1 : Inport
  Enable : EnablePort
  " " : MATLAB Function  TreatAsAtomicUnit=on
  Bus Creator : BusCreator  Inputs=3
  Bus Selector2 : BusSelector  OutputSignals=Point.X,Point.Y,Point.Z
  Out1 : Outport
  wires:
  Bus Creator/1 -> Out1/1
  In1/1 -> Bus Selector2/1
  Bus Selector2/2 -> " "/2(Y)  "<Y>"
  Bus Selector2/1 -> " "/1(X)  "<X>"
  " "/1(ang_x) -> Bus Creator/1
  " "/2(ang_y) -> Bus Creator/2
  " "/3(ang_z) -> Bus Creator/3
  Bus Selector2/3 -> " "/3(Z)  "<Z>"

== system fourBebop_circle/ang3 ==
  In1 : Inport
  Enable : EnablePort
  " " : MATLAB Function  TreatAsAtomicUnit=on
  Bus Creator : BusCreator  Inputs=3
  Bus Selector2 : BusSelector  OutputSignals=Point.X,Point.Y,Point.Z
  Out1 : Outport
  wires:
  Bus Creator/1 -> Out1/1
  In1/1 -> Bus Selector2/1
  Bus Selector2/2 -> " "/2(Y)  "<Y>"
  Bus Selector2/1 -> " "/1(X)  "<X>"
  " "/1(ang_x) -> Bus Creator/1
  " "/2(ang_y) -> Bus Creator/2
  " "/3(ang_z) -> Bus Creator/3
  Bus Selector2/3 -> " "/3(Z)  "<Z>"

== system fourBebop_circle/ang4 ==
  In1 : Inport
  Enable : EnablePort
  " " : MATLAB Function  TreatAsAtomicUnit=on
  Bus Creator : BusCreator  Inputs=3
  Bus Selector2 : BusSelector  OutputSignals=Point.X,Point.Y,Point.Z
  Out1 : Outport
  wires:
  Bus Creator/1 -> Out1/1
  In1/1 -> Bus Selector2/1
  Bus Selector2/2 -> " "/2(Y)  "<Y>"
  Bus Selector2/1 -> " "/1(X)  "<X>"
  " "/1(ang_x) -> Bus Creator/1
  " "/2(ang_y) -> Bus Creator/2
  " "/3(ang_z) -> Bus Creator/3
  Bus Selector2/3 -> " "/3(Z)  "<Z>"

== system fourBebop_circle/pos1 ==
  In1 : Inport
  Enable : EnablePort
  " " : MATLAB Function  TreatAsAtomicUnit=on
  Bus Creator : BusCreator  Inputs=3
  Bus Selector1 : BusSelector  OutputSignals=Point.X,Point.Y,Point.Z
  Out1 : Outport
  wires:
  Bus Creator/1 -> Out1/1
  In1/1 -> Bus Selector1/1
  Bus Selector1/1 -> " "/1(vps_X)  "<X>"
  Bus Selector1/2 -> " "/2(vps_Y)  "<Y>"
  Bus Selector1/3 -> " "/3(vps_Z)  "<Z>"
  " "/1(vps_x) -> Bus Creator/1
  " "/2(vps_y) -> Bus Creator/2
  " "/3(vps_z) -> Bus Creator/3

== system fourBebop_circle/pos2 ==
  In1 : Inport
  Enable : EnablePort
  " " : MATLAB Function  TreatAsAtomicUnit=on
  Bus Creator : BusCreator  Inputs=3
  Bus Selector1 : BusSelector  OutputSignals=Point.X,Point.Y,Point.Z
  Out1 : Outport
  wires:
  Bus Creator/1 -> Out1/1
  In1/1 -> Bus Selector1/1
  Bus Selector1/1 -> " "/1(vps_X)  "<X>"
  Bus Selector1/2 -> " "/2(vps_Y)  "<Y>"
  Bus Selector1/3 -> " "/3(vps_Z)  "<Z>"
  " "/1(vps_x) -> Bus Creator/1
  " "/2(vps_y) -> Bus Creator/2
  " "/3(vps_z) -> Bus Creator/3

== system fourBebop_circle/pos3 ==
  In1 : Inport
  Enable : EnablePort
  " " : MATLAB Function  TreatAsAtomicUnit=on
  Bus Creator : BusCreator  Inputs=3
  Bus Selector1 : BusSelector  OutputSignals=Point.X,Point.Y,Point.Z
  Out1 : Outport
  wires:
  Bus Creator/1 -> Out1/1
  In1/1 -> Bus Selector1/1
  Bus Selector1/1 -> " "/1(vps_X)  "<X>"
  Bus Selector1/2 -> " "/2(vps_Y)  "<Y>"
  Bus Selector1/3 -> " "/3(vps_Z)  "<Z>"
  " "/1(vps_x) -> Bus Creator/1
  " "/2(vps_y) -> Bus Creator/2
  " "/3(vps_z) -> Bus Creator/3

== system fourBebop_circle/pos4 ==
  In1 : Inport
  Enable : EnablePort
  " " : MATLAB Function  TreatAsAtomicUnit=on
  Bus Creator : BusCreator  Inputs=3
  Bus Selector1 : BusSelector  OutputSignals=Point.X,Point.Y,Point.Z
  Out1 : Outport
  wires:
  Bus Creator/1 -> Out1/1
  In1/1 -> Bus Selector1/1
  Bus Selector1/1 -> " "/1(vps_X)  "<X>"
  Bus Selector1/2 -> " "/2(vps_Y)  "<Y>"
  Bus Selector1/3 -> " "/3(vps_Z)  "<Z>"
  " "/1(vps_x) -> Bus Creator/1
  " "/2(vps_y) -> Bus Creator/2
  " "/3(vps_z) -> Bus Creator/3

== system fourBebop_circle/vel ==
  In1 : Inport
  Enable : EnablePort
  " 2" : MATLAB Function  TreatAsAtomicUnit=on
  Bus Creator : BusCreator  Inputs=3
  Bus Selector2 : BusSelector  OutputSignals=Twist.Linear.X,Twist.Linear.Y,Twist.Linear.Z
  Out1 : Outport
  wires:
  In1/1 -> Bus Selector2/1
  Bus Creator/1 -> Out1/1
  Bus Selector2/1 -> " 2"/1(vps_X)  "<X>"
  Bus Selector2/2 -> " 2"/2(vps_Y)  "<Y>"
  Bus Selector2/3 -> " 2"/3(vps_Z)  "<Z>"
  " 2"/1(vps_vx) -> Bus Creator/1
  " 2"/2(vps_vy) -> Bus Creator/2
  " 2"/3(vps_vz) -> Bus Creator/3

== system fourBebop_circle/vel1 ==
  In1 : Inport
  Enable : EnablePort
  " 2" : MATLAB Function  TreatAsAtomicUnit=on
  Bus Creator : BusCreator  Inputs=3
  Bus Selector2 : BusSelector  OutputSignals=Twist.Linear.X,Twist.Linear.Y,Twist.Linear.Z
  Out1 : Outport
  wires:
  In1/1 -> Bus Selector2/1
  Bus Creator/1 -> Out1/1
  Bus Selector2/1 -> " 2"/1(vps_X)  "<X>"
  Bus Selector2/2 -> " 2"/2(vps_Y)  "<Y>"
  Bus Selector2/3 -> " 2"/3(vps_Z)  "<Z>"
  " 2"/1(vps_vx) -> Bus Creator/1
  " 2"/2(vps_vy) -> Bus Creator/2
  " 2"/3(vps_vz) -> Bus Creator/3

== system fourBebop_circle/vel2 ==
  In1 : Inport
  Enable : EnablePort
  " 2" : MATLAB Function  TreatAsAtomicUnit=on
  Bus Creator : BusCreator  Inputs=3
  Bus Selector2 : BusSelector  OutputSignals=Twist.Linear.X,Twist.Linear.Y,Twist.Linear.Z
  Out1 : Outport
  wires:
  In1/1 -> Bus Selector2/1
  Bus Creator/1 -> Out1/1
  Bus Selector2/1 -> " 2"/1(vps_X)  "<X>"
  Bus Selector2/2 -> " 2"/2(vps_Y)  "<Y>"
  Bus Selector2/3 -> " 2"/3(vps_Z)  "<Z>"
  " 2"/1(vps_vx) -> Bus Creator/1
  " 2"/2(vps_vy) -> Bus Creator/2
  " 2"/3(vps_vz) -> Bus Creator/3

== system fourBebop_circle/vel3 ==
  In1 : Inport
  Enable : EnablePort
  " 2" : MATLAB Function  TreatAsAtomicUnit=on
  Bus Creator : BusCreator  Inputs=3
  Bus Selector2 : BusSelector  OutputSignals=Twist.Linear.X,Twist.Linear.Y,Twist.Linear.Z
  Out1 : Outport
  wires:
  In1/1 -> Bus Selector2/1
  Bus Creator/1 -> Out1/1
  Bus Selector2/1 -> " 2"/1(vps_X)  "<X>"
  Bus Selector2/2 -> " 2"/2(vps_Y)  "<Y>"
  Bus Selector2/3 -> " 2"/3(vps_Z)  "<Z>"
  " 2"/1(vps_vx) -> Bus Creator/1
  " 2"/2(vps_vy) -> Bus Creator/2
  " 2"/3(vps_vz) -> Bus Creator/3

== system fourBebop_circle/Baseline Controller1/Heading controller ==
  yaw_e (rad) : Inport
  yaw_d. (rad) : Inport  Port=2
  Sum1 : Sum  Inputs=|-+
  proportional control gain - yaw : Gain  Gain=0.5
  yaw_rate_d. (rad/s) : Outport
  wires:
  Sum1/1 -> proportional control gain - yaw/1
  proportional control gain - yaw/1 -> yaw_rate_d. (rad/s)/1
  yaw_e (rad)/1 -> Sum1/1
  yaw_d. (rad)/1 -> Sum1/2

== system fourBebop_circle/Baseline Controller1/Height controller  ==
  Z_d. (m) : Inport
  Z_e (m) : Inport  Port=2
  Sum3 : Sum  Inputs=|-+
  proportional control gain : Gain  Gain=0.5
  Z_velocity_d (m/s) : Outport
  wires:
  proportional control gain/1 -> Z_velocity_d (m/s)/1
  Sum3/1 -> proportional control gain/1
  Z_e (m)/1 -> Sum3/1
  Z_d. (m)/1 -> Sum3/2

== system fourBebop_circle/Baseline Controller1/Position controller ==
  X_e (m) : Inport
  Y_e (m) : Inport  Port=2
  Yaw_e (rad) : Inport  Port=3
  X_d (m) : Inport  Port=4
  Y_d (m) : Inport  Port=5
  "Coordinate trnasformation from inertial frame to body frame " : MATLAB Function  TreatAsAtomicUnit=on
  Demux : Demux  Outputs=2
  Gain2 : Gain  Gain=0.5
  Gain3 : Gain  Gain=0.5
  Mux : Mux  Inputs=2
  Mux1 : Mux  Inputs=2
  Sum4 : Sum  Inputs=|-+
  forward(x)_velocity_d. (m/s) : Outport
  lateral(y)_velocity_ref. (m/s) : Outport  Port=2
  wires:
  Gain2/1 -> forward(x)_velocity_d. (m/s)/1
  Yaw_e (rad)/1 -> "Coordinate trnasformation from inertial frame to body frame "/2(psi)
  "Coordinate trnasformation from inertial frame to body frame "/1(Vec_xy) -> Demux/1
  Mux1/1 -> Sum4/2
  Sum4/1 -> "Coordinate trnasformation from inertial frame to body frame "/1(Vec_i)
  Y_e (m)/1 -> Mux/2
  X_e (m)/1 -> Mux/1
  Mux/1 -> Sum4/1
  Demux/1 -> Gain2/1
  Demux/2 -> Gain3/1
  Gain3/1 -> lateral(y)_velocity_ref. (m/s)/1
  X_d (m)/1 -> Mux1/1
  Y_d (m)/1 -> Mux1/2

== system fourBebop_circle/Baseline Controller2/Heading controller ==
  yaw_e (rad) : Inport
  yaw_d. (rad) : Inport  Port=2
  Sum1 : Sum  Inputs=|-+
  proportional control gain - yaw : Gain  Gain=0.5
  yaw_rate_d. (rad/s) : Outport
  wires:
  Sum1/1 -> proportional control gain - yaw/1
  proportional control gain - yaw/1 -> yaw_rate_d. (rad/s)/1
  yaw_e (rad)/1 -> Sum1/1
  yaw_d. (rad)/1 -> Sum1/2

== system fourBebop_circle/Baseline Controller2/Height controller  ==
  Z_d. (m) : Inport
  Z_e (m) : Inport  Port=2
  Sum3 : Sum  Inputs=|-+
  proportional control gain : Gain  Gain=0.5
  Z_velocity_d (m/s) : Outport
  wires:
  proportional control gain/1 -> Z_velocity_d (m/s)/1
  Sum3/1 -> proportional control gain/1
  Z_e (m)/1 -> Sum3/1
  Z_d. (m)/1 -> Sum3/2

== system fourBebop_circle/Baseline Controller2/Position controller ==
  X_e (m) : Inport
  Y_e (m) : Inport  Port=2
  Yaw_e (rad) : Inport  Port=3
  X_d (m) : Inport  Port=4
  Y_d (m) : Inport  Port=5
  "Coordinate trnasformation from inertial frame to body frame " : MATLAB Function  TreatAsAtomicUnit=on
  Demux : Demux  Outputs=2
  Gain2 : Gain  Gain=0.5
  Gain3 : Gain  Gain=0.5
  Mux : Mux  Inputs=2
  Mux1 : Mux  Inputs=2
  Sum4 : Sum  Inputs=|-+
  forward(x)_velocity_d. (m/s) : Outport
  lateral(y)_velocity_ref. (m/s) : Outport  Port=2
  wires:
  Gain2/1 -> forward(x)_velocity_d. (m/s)/1
  Yaw_e (rad)/1 -> "Coordinate trnasformation from inertial frame to body frame "/2(psi)
  "Coordinate trnasformation from inertial frame to body frame "/1(Vec_xy) -> Demux/1
  Mux1/1 -> Sum4/2
  Sum4/1 -> "Coordinate trnasformation from inertial frame to body frame "/1(Vec_i)
  Y_e (m)/1 -> Mux/2
  X_e (m)/1 -> Mux/1
  Mux/1 -> Sum4/1
  Demux/1 -> Gain2/1
  Demux/2 -> Gain3/1
  Gain3/1 -> lateral(y)_velocity_ref. (m/s)/1
  X_d (m)/1 -> Mux1/1
  Y_d (m)/1 -> Mux1/2

== system fourBebop_circle/Baseline Controller3/Heading controller ==
  yaw_e (rad) : Inport
  yaw_d. (rad) : Inport  Port=2
  Sum1 : Sum  Inputs=|-+
  proportional control gain - yaw : Gain  Gain=0.5
  yaw_rate_d. (rad/s) : Outport
  wires:
  Sum1/1 -> proportional control gain - yaw/1
  proportional control gain - yaw/1 -> yaw_rate_d. (rad/s)/1
  yaw_e (rad)/1 -> Sum1/1
  yaw_d. (rad)/1 -> Sum1/2

== system fourBebop_circle/Baseline Controller3/Height controller  ==
  Z_d. (m) : Inport
  Z_e (m) : Inport  Port=2
  Sum3 : Sum  Inputs=|-+
  proportional control gain : Gain  Gain=0.5
  Z_velocity_d (m/s) : Outport
  wires:
  proportional control gain/1 -> Z_velocity_d (m/s)/1
  Sum3/1 -> proportional control gain/1
  Z_e (m)/1 -> Sum3/1
  Z_d. (m)/1 -> Sum3/2

== system fourBebop_circle/Baseline Controller3/Position controller ==
  X_e (m) : Inport
  Y_e (m) : Inport  Port=2
  Yaw_e (rad) : Inport  Port=3
  X_d (m) : Inport  Port=4
  Y_d (m) : Inport  Port=5
  "Coordinate trnasformation from inertial frame to body frame " : MATLAB Function  TreatAsAtomicUnit=on
  Demux : Demux  Outputs=2
  Gain2 : Gain  Gain=0.5
  Gain3 : Gain  Gain=0.5
  Mux : Mux  Inputs=2
  Mux1 : Mux  Inputs=2
  Sum4 : Sum  Inputs=|-+
  forward(x)_velocity_d. (m/s) : Outport
  lateral(y)_velocity_ref. (m/s) : Outport  Port=2
  wires:
  Gain2/1 -> forward(x)_velocity_d. (m/s)/1
  Yaw_e (rad)/1 -> "Coordinate trnasformation from inertial frame to body frame "/2(psi)
  "Coordinate trnasformation from inertial frame to body frame "/1(Vec_xy) -> Demux/1
  Mux1/1 -> Sum4/2
  Sum4/1 -> "Coordinate trnasformation from inertial frame to body frame "/1(Vec_i)
  Y_e (m)/1 -> Mux/2
  X_e (m)/1 -> Mux/1
  Mux/1 -> Sum4/1
  Demux/1 -> Gain2/1
  Demux/2 -> Gain3/1
  Gain3/1 -> lateral(y)_velocity_ref. (m/s)/1
  X_d (m)/1 -> Mux1/1
  Y_d (m)/1 -> Mux1/2

== system fourBebop_circle/Baseline Controller4/Heading controller ==
  yaw_e (rad) : Inport
  yaw_d. (rad) : Inport  Port=2
  Sum1 : Sum  Inputs=|-+
  proportional control gain - yaw : Gain  Gain=0.5
  yaw_rate_d. (rad/s) : Outport
  wires:
  Sum1/1 -> proportional control gain - yaw/1
  proportional control gain - yaw/1 -> yaw_rate_d. (rad/s)/1
  yaw_e (rad)/1 -> Sum1/1
  yaw_d. (rad)/1 -> Sum1/2

== system fourBebop_circle/Baseline Controller4/Height controller  ==
  Z_d. (m) : Inport
  Z_e (m) : Inport  Port=2
  Sum3 : Sum  Inputs=|-+
  proportional control gain : Gain  Gain=0.5
  Z_velocity_d (m/s) : Outport
  wires:
  proportional control gain/1 -> Z_velocity_d (m/s)/1
  Sum3/1 -> proportional control gain/1
  Z_e (m)/1 -> Sum3/1
  Z_d. (m)/1 -> Sum3/2

== system fourBebop_circle/Baseline Controller4/Position controller ==
  X_e (m) : Inport
  Y_e (m) : Inport  Port=2
  Yaw_e (rad) : Inport  Port=3
  X_d (m) : Inport  Port=4
  Y_d (m) : Inport  Port=5
  "Coordinate trnasformation from inertial frame to body frame " : MATLAB Function  TreatAsAtomicUnit=on
  Demux : Demux  Outputs=2
  Gain2 : Gain  Gain=0.5
  Gain3 : Gain  Gain=0.5
  Mux : Mux  Inputs=2
  Mux1 : Mux  Inputs=2
  Sum4 : Sum  Inputs=|-+
  forward(x)_velocity_d. (m/s) : Outport
  lateral(y)_velocity_ref. (m/s) : Outport  Port=2
  wires:
  Gain2/1 -> forward(x)_velocity_d. (m/s)/1
  Yaw_e (rad)/1 -> "Coordinate trnasformation from inertial frame to body frame "/2(psi)
  "Coordinate trnasformation from inertial frame to body frame "/1(Vec_xy) -> Demux/1
  Mux1/1 -> Sum4/2
  Sum4/1 -> "Coordinate trnasformation from inertial frame to body frame "/1(Vec_i)
  Y_e (m)/1 -> Mux/2
  X_e (m)/1 -> Mux/1
  Mux/1 -> Sum4/1
  Demux/1 -> Gain2/1
  Demux/2 -> Gain3/1
  Gain3/1 -> lateral(y)_velocity_ref. (m/s)/1
  X_d (m)/1 -> Mux1/1
  Y_d (m)/1 -> Mux1/2

== matlab function fourBebop_circle/MATLAB Function ==
  data: u input; y output; lostsigalcount input
function y = fcn(u,lostsigalcount)


if  -0.00001<u & u<0.00001
    lostsigalcount = lostsigalcount +1;
else
    lostsigalcount = 0;
end

if lostsigalcount>=3
  y=0;
else
  y=1;
end

== matlab function fourBebop_circle/ang1/  ==
  data: ang_x output; X input; ang_y output; Y input; Z input; ang_z output
function [ang_x, ang_y, ang_z] = angle_tf(X, Y, Z)
ang_x =  X*pi/180;
ang_y =  -Y*pi/180;
ang_z =  -Z*pi/180;

== matlab function fourBebop_circle/Baseline Controller1/MATLAB Function ==
  data: u input; y output; a input
function y = fcn(u,a)
y = satgd(u,a);

== matlab function fourBebop_circle/Baseline Controller2/MATLAB Function ==
  data: u input; y output; a input
function y = fcn(u,a)
y = satgd(u,a);

== matlab function fourBebop_circle/pos1/  ==
  data: vps_x output; vps_X input; vps_y output; vps_Y input; vps_Z input; vps_z output
function [vps_x, vps_y, vps_z] = xyz_offset(vps_X, vps_Y, vps_Z)
% x =  vps_X + offset_X;
% y =  -vps_Y+offset_Y;
% z =  vps_Z+offset_Z;
temp=[vps_X;vps_Y;vps_Z];
vps_x=temp(1);
vps_y=temp(2);
vps_z=temp(3);

== matlab function fourBebop_circle/Baseline Controller2/Position controller/Coordinate trnasformation from inertial frame to body frame  ==
  data: Vec_i input; Vec_xy output; psi input
function Vec_xy  = fcn(Vec_i , psi)
%#codegen
T = [cos(psi) sin(psi) ; -sin(psi) cos(psi)] ; 
Vec_xy = T*Vec_i(1:2,1);

== matlab function fourBebop_circle/Baseline Controller1/Position controller/Coordinate trnasformation from inertial frame to body frame  ==
  data: Vec_i input; Vec_xy output; psi input
function Vec_xy  = fcn(Vec_i , psi)
%#codegen
T = [cos(psi) sin(psi) ; -sin(psi) cos(psi)] ; 
Vec_xy = T*Vec_i(1:2,1);

== matlab function fourBebop_circle/MATLAB Function1 ==
  data: u input; y output; lostsigalcount input
function y = fcn(u,lostsigalcount)


if  -0.00001<u & u<0.00001
    lostsigalcount = lostsigalcount +1;
else
    lostsigalcount = 0;
end

if lostsigalcount>=3
  y=0;
else
  y=1;
end

== matlab function fourBebop_circle/ang2/  ==
  data: ang_x output; X input; ang_y output; Y input; Z input; ang_z output
function [ang_x, ang_y, ang_z] = angle_tf(X, Y, Z)
ang_x =  X*pi/180;
ang_y =  -Y*pi/180;
ang_z =  -Z*pi/180;

== matlab function fourBebop_circle/vel/ 2 ==
  data: vps_vx output; vps_X input; vps_vy output; vps_Y input; vps_Z input; vps_vz output
function [vps_vx, vps_vy, vps_vz] = vxyz_offset(vps_X, vps_Y, vps_Z)
% x =  vps_X + offset_X;
% y =  -vps_Y+offset_Y;
% z =  vps_Z+offset_Z;
temp=[vps_X;vps_Y;vps_Z];
vps_vx=temp(1);
vps_vy=temp(2);
vps_vz=temp(3);

== matlab function fourBebop_circle/pos2/  ==
  data: vps_x output; vps_X input; vps_y output; vps_Y input; vps_Z input; vps_z output
function [vps_x, vps_y, vps_z] = xyz_offset(vps_X, vps_Y, vps_Z)
% x =  vps_X + offset_X;
% y =  -vps_Y+offset_Y;
% z =  vps_Z+offset_Z;
temp=[vps_X;vps_Y;vps_Z];
vps_x=temp(1);
vps_y=temp(2);
vps_z=temp(3);

== matlab function fourBebop_circle/vel2/ 2 ==
  data: vps_vx output; vps_X input; vps_vy output; vps_Y input; vps_Z input; vps_vz output
function [vps_vx, vps_vy, vps_vz] = vxyz_offset(vps_X, vps_Y, vps_Z)
% x =  vps_X + offset_X;
% y =  -vps_Y+offset_Y;
% z =  vps_Z+offset_Z;
temp=[vps_X;vps_Y;vps_Z];
vps_vx=temp(1);
vps_vy=temp(2);
vps_vz=temp(3);

== matlab function fourBebop_circle/Baseline Controller3/MATLAB Function ==
  data: u input; y output; a input
function y = fcn(u,a)
y = satgd(u,a);

== matlab function fourBebop_circle/Baseline Controller3/Position controller/Coordinate trnasformation from inertial frame to body frame  ==
  data: Vec_i input; Vec_xy output; psi input
function Vec_xy  = fcn(Vec_i , psi)
%#codegen
T = [cos(psi) sin(psi) ; -sin(psi) cos(psi)] ; 
Vec_xy = T*Vec_i(1:2,1);

== matlab function fourBebop_circle/MATLAB Function2 ==
  data: u input; y output; lostsigalcount input
function y = fcn(u,lostsigalcount)


if  -0.00001<u & u<0.00001
    lostsigalcount = lostsigalcount +1;
else
    lostsigalcount = 0;
end

if lostsigalcount>=3
  y=0;
else
  y=1;
end

== matlab function fourBebop_circle/ang3/  ==
  data: ang_x output; X input; ang_y output; Y input; Z input; ang_z output
function [ang_x, ang_y, ang_z] = angle_tf(X, Y, Z)
ang_x =  X*pi/180;
ang_y =  -Y*pi/180;
ang_z =  -Z*pi/180;

== matlab function fourBebop_circle/pos3/  ==
  data: vps_x output; vps_X input; vps_y output; vps_Y input; vps_Z input; vps_z output
function [vps_x, vps_y, vps_z] = xyz_offset(vps_X, vps_Y, vps_Z)
% x =  vps_X + offset_X;
% y =  -vps_Y+offset_Y;
% z =  vps_Z+offset_Z;
temp=[vps_X;vps_Y;vps_Z];
vps_x=temp(1);
vps_y=temp(2);
vps_z=temp(3);

== matlab function fourBebop_circle/vel1/ 2 ==
  data: vps_vx output; vps_X input; vps_vy output; vps_Y input; vps_Z input; vps_vz output
function [vps_vx, vps_vy, vps_vz] = vxyz_offset(vps_X, vps_Y, vps_Z)
% x =  vps_X + offset_X;
% y =  -vps_Y+offset_Y;
% z =  vps_Z+offset_Z;
temp=[vps_X;vps_Y;vps_Z];
vps_vx=temp(1);
vps_vy=temp(2);
vps_vz=temp(3);
